simulink model "sys_PID"  (R2021a)
settings: Solver=FixedStepAuto  StartTime=0.0  StopTime=500  FixedStep=0.02  RelTol=1e-3
libraries: sharedutil x5, simulink x3, aerolibutil x1
(part 1 of 2)
settings Model: Creator=frede  LastModifiedBy=frede
settings DataIOCC: ReturnWorkspaceOutputs=off

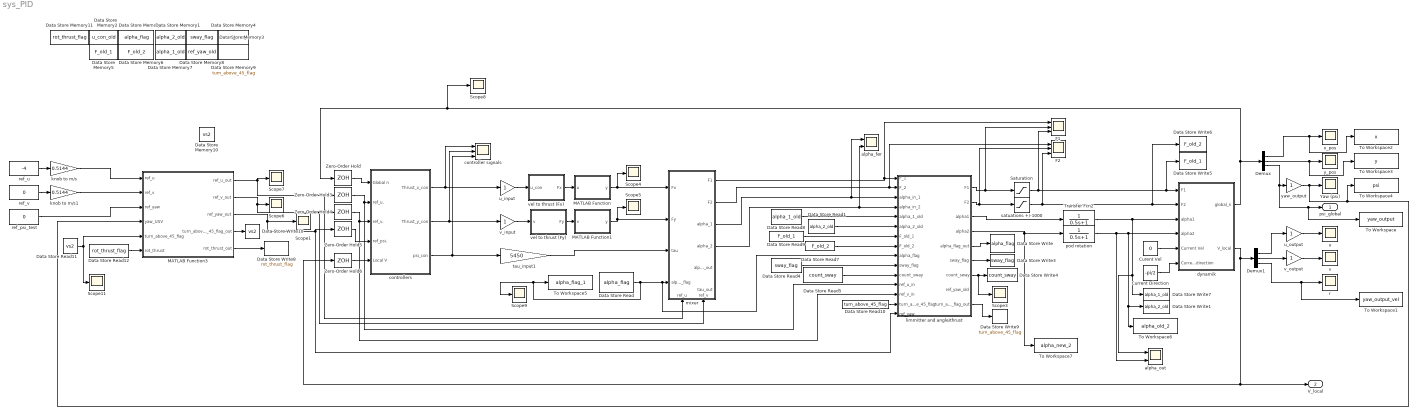
== system sys_PID ==
  Curent Vel : Constant  Value=0
  Current Direction : Constant  Value=-pi/2
  Data Store Memory : DataStoreMemory  DataStoreName=alpha_flag  ReadBeforeWriteMsg=warning  WriteAfterWriteMsg=warning  WriteAfterReadMsg=warning  ShowAdditionalParam=off
  Data Store Memory1 : DataStoreMemory  DataStoreName=alpha_2_old  ReadBeforeWriteMsg=warning  WriteAfterWriteMsg=warning  WriteAfterReadMsg=warning  ShowAdditionalParam=off
  Data Store Memory10 : DataStoreMemory  DataStoreName=vs2  ReadBeforeWriteMsg=warning  WriteAfterWriteMsg=warning  WriteAfterReadMsg=warning  ShowAdditionalParam=off
  Data Store Memory11 : DataStoreMemory  DataStoreName=rot_thrust_flag  ReadBeforeWriteMsg=warning  WriteAfterWriteMsg=warning  WriteAfterReadMsg=warning  ShowAdditionalParam=off
  Data Store Memory2 : DataStoreMemory  DataStoreName=u_con_old  ReadBeforeWriteMsg=warning  WriteAfterWriteMsg=warning  WriteAfterReadMsg=warning  ShowAdditionalParam=off
  Data Store Memory3 : DataStoreMemory  DataStoreName=sway_flag  ReadBeforeWriteMsg=warning  WriteAfterWriteMsg=warning  WriteAfterReadMsg=warning  ShowAdditionalParam=off
  Data Store Memory4 : DataStoreMemory  DataStoreName=count_sway  ReadBeforeWriteMsg=warning  WriteAfterWriteMsg=warning  WriteAfterReadMsg=warning  ShowAdditionalParam=off
  Data Store Memory5 : DataStoreMemory  DataStoreName=F_old_1  ReadBeforeWriteMsg=warning  WriteAfterWriteMsg=warning  WriteAfterReadMsg=warning  ShowAdditionalParam=off
  Data Store Memory6 : DataStoreMemory  DataStoreName=F_old_2  ReadBeforeWriteMsg=warning  WriteAfterWriteMsg=warning  WriteAfterReadMsg=warning  ShowAdditionalParam=off
  Data Store Memory7 : DataStoreMemory  DataStoreName=alpha_1_old  ReadBeforeWriteMsg=warning  WriteAfterWriteMsg=warning  WriteAfterReadMsg=warning  ShowAdditionalParam=off
  Data Store Memory8 : DataStoreMemory  DataStoreName=ref_yaw_old  ReadBeforeWriteMsg=warning  WriteAfterWriteMsg=warning  WriteAfterReadMsg=warning  ShowAdditionalParam=off
  Data Store Memory9 : DataStoreMemory  DataStoreName=turn_above_45_flag  ReadBeforeWriteMsg=warning  WriteAfterWriteMsg=warning  WriteAfterReadMsg=warning  ShowAdditionalParam=off
  Data Store Read : DataStoreRead  DataStoreName=alpha_flag  IndexOptions=Index vector (dialog)  Indices=1  OutputSizes=1
  Data Store Read1 : DataStoreRead  DataStoreName=alpha_2_old  IndexOptions=Index vector (dialog)  Indices=1  OutputSizes=1
  Data Store Read10 : DataStoreRead  DataStoreName=turn_above_45_flag  IndexOptions=Index vector (dialog)  Indices=1  OutputSizes=1
  Data Store Read11 : DataStoreRead  DataStoreName=vs2  IndexOptions=Index vector (dialog)  Indices=1  OutputSizes=1
  Data Store Read12 : DataStoreRead  DataStoreName=rot_thrust_flag  IndexOptions=Index vector (dialog)  Indices=1  OutputSizes=1
  Data Store Read4 : DataStoreRead  DataStoreName=sway_flag  IndexOptions=Index vector (dialog)  Indices=1  OutputSizes=1
  Data Store Read5 : DataStoreRead  DataStoreName=count_sway  IndexOptions=Index vector (dialog)  Indices=1  OutputSizes=1
  Data Store Read7 : DataStoreRead  DataStoreName=F_old_2  IndexOptions=Index vector (dialog)  Indices=1  OutputSizes=1
  Data Store Read8 : DataStoreRead  DataStoreName=alpha_1_old  IndexOptions=Index vector (dialog)  Indices=1  OutputSizes=1
  Data Store Read9 : DataStoreRead  DataStoreName=F_old_1  IndexOptions=Index vector (dialog)  Indices=1  OutputSizes=1
  Data Store Write : DataStoreWrite  DataStoreName=alpha_flag  IndexOptions=Index vector (dialog)  Indices=1  OutputSizes=1
  Data Store Write1 : DataStoreWrite  DataStoreName=alpha_2_old  IndexOptions=Index vector (dialog)  Indices=1  OutputSizes=1
  Data Store Write10 : DataStoreWrite  DataStoreName=vs2  IndexOptions=Index vector (dialog)  Indices=1  OutputSizes=1
  Data Store Write3 : DataStoreWrite  DataStoreName=sway_flag  IndexOptions=Index vector (dialog)  Indices=1  OutputSizes=1
  Data Store Write4 : DataStoreWrite  DataStoreName=count_sway  IndexOptions=Index vector (dialog)  Indices=1  OutputSizes=1
  Data Store Write5 : DataStoreWrite  DataStoreName=F_old_1  IndexOptions=Index vector (dialog)  Indices=1  OutputSizes=1
  Data Store Write6 : DataStoreWrite  DataStoreName=F_old_2  IndexOptions=Index vector (dialog)  Indices=1  OutputSizes=1
  Data Store Write7 : DataStoreWrite  DataStoreName=alpha_1_old  IndexOptions=Index vector (dialog)  Indices=1  OutputSizes=1
  Data Store Write8 : DataStoreWrite  DataStoreName=rot_thrust_flag  IndexOptions=Index vector (dialog)  Indices=1  OutputSizes=1
  Data Store Write9 : DataStoreWrite  DataStoreName=turn_above_45_flag  IndexOptions=Index vector (dialog)  Indices=1  OutputSizes=1
  Demux : Demux  Outputs=3
  Demux1 : Demux  Outputs=3
  F1 : Scope  NumInputPorts=3
  F2 : Scope  NumInputPorts=3
  MATLAB Function : MATLAB Function  TreatAsAtomicUnit=on
  MATLAB Function1 : MATLAB Function  TreatAsAtomicUnit=on
  MATLAB Function3 : MATLAB Function  TreatAsAtomicUnit=on
  Saturation : Saturate  UpperLimit=1000  LowerLimit=-1000
  Scope{1,3..9,11} (9 alike) : Scope
  To Workspace : ToWorkspace  VariableName=yaw_output  SaveFormat=Timeseries  SampleTime=-1
  To Workspace1 : ToWorkspace  VariableName=yaw_output_vel  SaveFormat=Timeseries  SampleTime=-1
  To Workspace2 : ToWorkspace  VariableName=x  SaveFormat=Timeseries  SampleTime=-1
  To Workspace3 : ToWorkspace  VariableName=y  SaveFormat=Timeseries  SampleTime=-1
  To Workspace4 : ToWorkspace  VariableName=psi  SaveFormat=Timeseries  SampleTime=-1
  To Workspace5 : ToWorkspace  VariableName=alpha_flag_1  SaveFormat=Timeseries  SampleTime=-1
  To Workspace6 : ToWorkspace  VariableName=alpha_old_2  SaveFormat=Timeseries  SampleTime=-1
  To Workspace7 : ToWorkspace  VariableName=alpha_new_2  SaveFormat=Timeseries  SampleTime=-1
  Transfer Fcn2 : TransferFcn  Denominator=[0.5 1]
  Yaw (psi) : Scope
  Zero-Order Hold{,3..6} (5 alike) : ZeroOrderHold  SampleTime=1/10
  alpha_før : Scope  NumInputPorts=2
  alpha_out : Scope  NumInputPorts=2
  controller signals : Scope  NumInputPorts=3
  controllers : Subsystem
  dynamik : Subsystem
  knob to m/s : Gain  Gain=0.5144
  knob to m/s1 : Gain  Gain=0.5144
  "limmitter and angle/thrust " : MATLAB Function  TreatAsAtomicUnit=on
  mixer : Subsystem
      settings: PortSchema="{\"entries\":[{\"content\":{\"sides\":[{\"content\":{\"connectorIds\":[\"In1\",\"In2\",\"In3\",\"In4\"]},\"type\":\"ConnectorPlacement.EquallySpacedRectSide\",\"uuid\":\"7188d02b-cfcc-47db-af94-18894173419c\"},{\"content\":{\"connectorIds\":[\"Out1\",\"Out2\",\"Out3\",\"Out4\",\"Out5\",\"Out6\"],\"side\":\"RIGHT\"},\"type\":\"ConnectorPlacement.EquallySpacedRectSide\",\"uuid\":\"02945fdb-bbe4-4a20-85bf-b896b72802e6\"},{\"content\":{\"connectorIds\":[],\"side\":\"TOP\"},\"type\":\"ConnectorPlacement.EquallySpacedRectSide\",\"uuid\":\"f10c450a-087c-46ba-bf6c-a28873fc7004\"},{\"content\":{\"connectorIds\":[\"In5\",\"In6\"],\"side\":\"BOTTOM\"},\"type\":\"ConnectorPlacement.EquallySpacedRectSide\",\"uuid\":\"e6b9d579-da5b-4e58-b3fd-82de45e53b4e\"}]},\"type\":\"ConnectorPlacement.EquallySpacedConnector\",\"uuid\":\"11fe65e6-3ea5-4662-a95f-67184bab7731\"}],\"packageUris\":[\"http://schema.mathworks.com/mf0/Connector/R2020b\"],\"version\":\"1.0\"}"
  pod rotation : TransferFcn  Denominator=[0.5 1]
  r : Scope
  ref_psi_test : Constant  Value=0
  ref_u : Constant  Value=-4
  ref_v : Constant  Value=0
  "satuations +/-1000 " : Saturate  UpperLimit=1000  LowerLimit=-1000
  tau_input1 : Gain  Gain=5450
  u : Scope
  u_input : Gain
  u_output : Gain
  v : Scope
  v_input : Gain
  v_output : Gain
  vel to thrust (Fx) : MATLAB Function  TreatAsAtomicUnit=on
  vel to thrust (Fy) : MATLAB Function  TreatAsAtomicUnit=on
  x_pos : Scope
  y_pos : Scope
  yaw_output : Gain
  psi_global : Outport
  V_local : Outport  Port=2
  wires:
  u_output/1 -> u/1
  vel to thrust (Fx)/1(Fx) -> MATLAB Function/1(u)
  Demux1/3 -> To Workspace1/1, r/1
  "limmitter and angle/thrust "/2(F2) -> "satuations +/-1000 "/1, F2/2
  mixer/1(F1) -> F1/1, "limmitter and angle/thrust "/1(F_1)
  v_input/1 -> vel to thrust (Fy)/1(v)
  pod rotation/1 -> dynamik/4(alpha2), To Workspace6/1, Data Store Write1/1, alpha_out/2
  mixer/4(alpha_2) -> alpha_før/2, "limmitter and angle/thrust "/4(alpha_in_2)
  Demux1/2 -> v_output/1
  mixer/2(F2) -> F2/1, "limmitter and angle/thrust "/2(F_2)
  "limmitter and angle/thrust "/3(alpha1) -> Transfer Fcn2/1
  u_input/1 -> vel to thrust (Fx)/1(u_con)
  MATLAB Function1/1(y) -> Scope5/1, mixer/2(Fy)
  mixer/3(alpha_1) -> alpha_før/1, "limmitter and angle/thrust "/3(alpha_in_1)
  "limmitter and angle/thrust "/1(F1) -> F1/2, Saturation/1
  Demux/2 -> To Workspace3/1, y_pos/1
  "satuations +/-1000 "/1 -> Data Store Write6/1, dynamik/2(F2), F2/3
  Demux1/1 -> u_output/1
  Transfer Fcn2/1 -> Data Store Write7/1, alpha_out/1, dynamik/3(alpha1)
  dynamik/1(global_n) -> Scope8/1, Zero-Order Hold/1, Demux/1
  "limmitter and angle/thrust "/4(alpha2) -> To Workspace7/1, pod rotation/1
  Demux/1 -> To Workspace2/1, x_pos/1
  v_output/1 -> v/1
  Saturation/1 -> Data Store Write5/1, dynamik/1(F1), F1/3
  ref_v/1 -> knob to m/s1/1
  Demux/3 -> yaw_output/1, To Workspace/1, psi_global/1
  MATLAB Function/1(y) -> Scope4/1, mixer/1(Fx)
  yaw_output/1 -> MATLAB Function3/4(yaw_USV), To Workspace4/1, Yaw (psi)/1
  vel to thrust (Fy)/1(Fy) -> MATLAB Function1/1(v)
  MATLAB Function3/3(ref_yaw_out) -> Zero-Order Hold5/1, "limmitter and angle/thrust "/15(ref_yaw), Scope1/1
  Curent Vel/1 -> dynamik/5(Current Vel)
  Current Direction/1 -> dynamik/6(Current direction)
  ref_u/1 -> knob to m/s/1
  MATLAB Function3/2(ref_v_out) -> Zero-Order Hold4/1, mixer/6(ref_v), Scope6/1
  "limmitter and angle/thrust "/5(alpha_flag_out) -> Data Store Write/1
  Data Store Read1/1 -> "limmitter and angle/thrust "/6(alpha_2_old)
  Data Store Read/1 -> Scope9/1, To Workspace5/1, "limmitter and angle/thrust "/9(alpha_flag), mixer/4(alpha_flag)
  Zero-Order Hold/1 -> controllers/1(Global n)
  MATLAB Function3/1(ref_u_out) -> Scope7/1, Zero-Order Hold3/1, mixer/5(ref_u)
  dynamik/2(V_local) -> Zero-Order Hold6/1, V_local/1, Demux1/1
  Zero-Order Hold3/1 -> "limmitter and angle/thrust "/12(ref_u_in), controllers/2(ref_u.)
  Zero-Order Hold4/1 -> controllers/3(ref_v.), "limmitter and angle/thrust "/13(ref_v_in)
  Zero-Order Hold5/1 -> controllers/4(ref_psi.)
  Zero-Order Hold6/1 -> controllers/5(Local V)
  "limmitter and angle/thrust "/6(sway_flag) -> Data Store Write3/1
  Data Store Read5/1 -> "limmitter and angle/thrust "/11("count_sway ")
  tau_input1/1 -> mixer/3(tau)
  Data Store Read8/1 -> "limmitter and angle/thrust "/5(alpha_1_old)
  Data Store Read7/1 -> "limmitter and angle/thrust "/8(F_old_2)
  Data Store Read9/1 -> "limmitter and angle/thrust "/7(F_old_1)
  Data Store Read4/1 -> "limmitter and angle/thrust "/10("sway_flag ")
  "limmitter and angle/thrust "/7(count_sway) -> Scope3/1, Data Store Write4/1
  Data Store Read10/1 -> "limmitter and angle/thrust "/14(turn_above_45_flag)
  "limmitter and angle/thrust "/9(turn_above_45_flag_out) -> Data Store Write9/1
  MATLAB Function3/4(turn_above_45_flag_out) -> Data Store Write10/1
  Data Store Read11/1 -> Scope11/1, MATLAB Function3/5(turn_above_45_flag)
  controllers/2(Thrust_y_con) -> v_input/1, controller signals/2
  controllers/1(Thrust_x_con) -> controller signals/1, u_input/1
  controllers/3(psi_con) -> tau_input1/1, controller signals/3
  Data Store Read12/1 -> MATLAB Function3/6(rot_thrust)
  MATLAB Function3/5(rot_thrust_out) -> Data Store Write8/1
  knob to m/s/1 -> MATLAB Function3/1(ref_u)
  knob to m/s1/1 -> MATLAB Function3/2(ref_v)
  ref_psi_test/1 -> MATLAB Function3/3(ref_yaw)

== system sys_PID/controllers ==
  Global n : Inport
  ref_u. : Inport  Port=2
  ref_v. : Inport  Port=3
  ref_psi. : Inport  Port=4
  Local V : Inport  Port=5
  PIDs : Subsystem
  Thrust_x_con : Outport
  Thrust_y_con : Outport  Port=2
  psi_con : Outport  Port=3
  wires:
  Global n/1 -> PIDs/1(n)
  ref_v./1 -> PIDs/4(ref_v_)
  PIDs/3(diff_psi) -> psi_con/1
  PIDs/1(sig_u) -> Thrust_x_con/1
  PIDs/2(sig_v) -> Thrust_y_con/1
  ref_u./1 -> PIDs/2(ref_u_)
  Local V/1 -> PIDs/3(V)
  ref_psi./1 -> PIDs/5(ref_psi_)

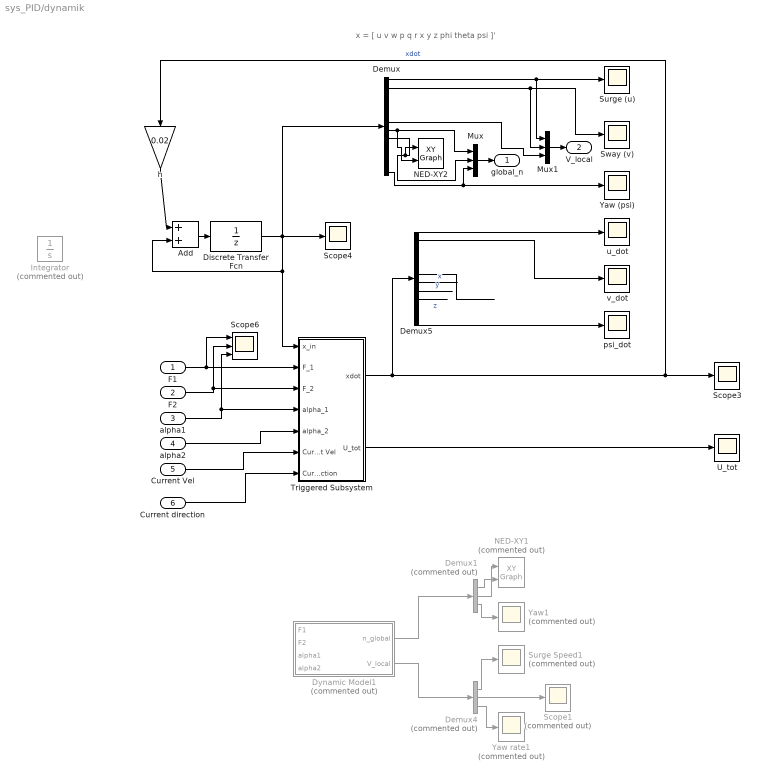
== system sys_PID/dynamik ==
  note: x = [ u v w p q r x y z phi theta psi ]'
  F1 : Inport
  F2 : Inport  Port=2
  alpha1 : Inport  Port=3
  alpha2 : Inport  Port=4
  Current Vel : Inport  Port=5
  Current direction : Inport  Port=6
  Add : Sum
  Demux : Demux  Outputs=12
  Demux1 : Demux  Commented=on  Outputs=3
  Demux4 : Demux  Commented=on  Outputs=3
  Demux5 : Demux  Outputs=12
  Discrete Transfer Fcn : DiscreteTransferFcn  Denominator=[ 1 0]  SampleTime=0.02
  Dynamic Model1 : Subsystem  Commented=on
  Integrator : Integrator  Commented=on
  Mux : Mux  Inputs=3
  Mux1 : Mux  Inputs=3
  NED-XY1 : simulink/Sinks/XY Graph  Commented=on  xmin=-1000  xmax=1000  ymin=-1000  ymax=1000  st=-1
  NED-XY2 : simulink/Sinks/XY Graph  xmin=-1000  xmax=1000  ymin=-1000  ymax=1000  st=-1
  Scope1 : Scope  Commented=on
  Scope3 : Scope
  Scope4 : Scope
  Scope6 : Scope  NumInputPorts=3
  Surge (u) : Scope
  Surge Speed1 : Scope  Commented=on
  Sway (v) : Scope
  Triggered Subsystem : Subsystem  TreatAsAtomicUnit=on
  U_tot : Scope
  Yaw (psi) : Scope
  Yaw rate1 : Scope  Commented=on
  Yaw1 : Scope  Commented=on
  h : Gain  Gain=0.02
  psi_dot : Scope
  u_dot : Scope
  v_dot : Scope
  global_n : Outport
  V_local : Outport  Port=2
  wires:
  Demux1/3 -> Yaw1/1
  Demux4/3 -> Yaw rate1/1
  Demux1/2 -> NED-XY1/1
  Demux4/2 -> Scope1/1
  Demux1/1 -> NED-XY1/2
  Demux4/1 -> Surge Speed1/1
  Dynamic Model1/1(n_global) -> Demux1/1
  Dynamic Model1/2(V_local) -> Demux4/1
  F1/1 -> Scope6/1, Triggered Subsystem/2(F_1)
  F2/1 -> Scope6/2, Triggered Subsystem/3(F_2)
  alpha1/1 -> Scope6/3, Triggered Subsystem/4(alpha_1)
  alpha2/1 -> Triggered Subsystem/5(alpha_2)
  h/1 -> Add/1
  Add/1 -> Discrete Transfer Fcn/1
  Triggered Subsystem/1(xdot) -> Demux5/1, Scope3/1, h/1  "xdot"
  Triggered Subsystem/2(U_tot) -> U_tot/1
  Demux/8 -> Mux/2, NED-XY2/1
  Demux/7 -> NED-XY2/2, Mux/1
  Discrete Transfer Fcn/1 -> Scope4/1, Demux/1, Add/2, Triggered Subsystem/1(x_in)
  Demux/1 -> Surge (u)/1, Mux1/1
  Demux/12 -> Mux/3, Yaw (psi)/1
  Demux/2 -> Mux1/2, Sway (v)/1
  Mux/1 -> global_n/1
  Demux5/12 -> psi_dot/1
  Demux5/2 -> v_dot/1
  Demux5/1 -> u_dot/1
  Demux5/9 -> ?  "z"
  Demux5/7 -> ?  "x"
  Demux5/8 -> ?  "y"
  Mux1/1 -> V_local/1
  Demux5/6 -> ?
  Demux/6 -> Mux1/3
  Current Vel/1 -> Triggered Subsystem/6(Current Vel)
  Current direction/1 -> Triggered Subsystem/7(Current Direction)

== system sys_PID/mixer ==
  Fx : Inport
  Fy : Inport  Port=2
  tau : Inport  Port=3
  alpha_flag : Inport  Port=4
  ref_u : Inport  Port=5
  ref_v : Inport  Port=6
  MATLAB Function : MATLAB Function  TreatAsAtomicUnit=on
  d : Constant  Value=1.3395
  F1 : Outport
  F2 : Outport  Port=2
  alpha_1 : Outport  Port=3
  alpha_2 : Outport  Port=4
  alpha_flag_out : Outport  Port=5
  tau_out : Outport  Port=6
  wires:
  d/1 -> MATLAB Function/4(d)
  MATLAB Function/1(F_1) -> F1/1
  Fx/1 -> MATLAB Function/1(F_x)
  Fy/1 -> MATLAB Function/2(F_y)
  tau/1 -> MATLAB Function/3(tau)
  MATLAB Function/2(F_2) -> F2/1
  MATLAB Function/3(alpha1) -> alpha_1/1
  MATLAB Function/4(alpha2) -> alpha_2/1
  alpha_flag/1 -> MATLAB Function/5(alpha_flag)
  MATLAB Function/5(alpha_flag_out) -> alpha_flag_out/1
  ref_u/1 -> MATLAB Function/7(ref_u)
  ref_v/1 -> MATLAB Function/8(ref_v)
  MATLAB Function/6(tau_out) -> tau_out/1

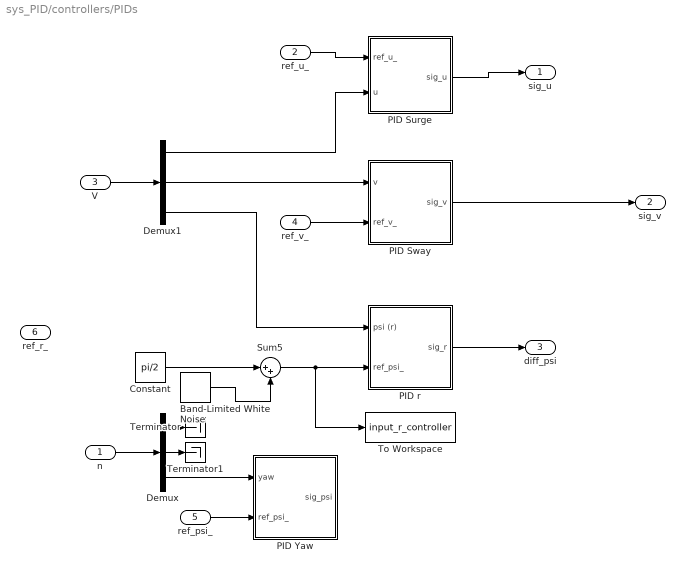
== system sys_PID/controllers/PIDs ==
  n : Inport
  ref_u_ : Inport  Port=2
  V : Inport  Port=3
  ref_v_ : Inport  Port=4
  ref_psi_ : Inport  Port=5
  ref_r_ : Inport  Port=6
  Band-Limited White Noise : simulink/Sources/Band-Limited White Noise  Cov=[0.01]  Ts=0.1  seed=[23341]
  Constant : Constant  Value=pi/2
  Demux : Demux  Outputs=3
  Demux1 : Demux  Outputs=3
  PID Surge : Subsystem
  PID Sway : Subsystem
  PID Yaw : Subsystem
  PID r : Subsystem
  Sum5 : Sum  Inputs=|++
  Terminator : Terminator
  Terminator1 : Terminator
  To Workspace : ToWorkspace  VariableName=input_r_controller  SaveFormat=Timeseries  SampleTime=-1
  sig_u : Outport
  sig_v : Outport  Port=2
  diff_psi : Outport  Port=3
  wires:
  n/1 -> Demux/1
  Demux/3 -> PID Yaw/1(yaw)
  Demux/1 -> Terminator/1
  Demux/2 -> Terminator1/1
  Demux1/3 -> PID r/1(psi (r))
  V/1 -> Demux1/1
  ref_u_/1 -> PID Surge/1(ref_u_)
  Demux1/1 -> PID Surge/2(u)
  Demux1/2 -> PID Sway/1(v)
  ref_v_/1 -> PID Sway/2(ref_v_)
  Band-Limited White Noise/1 -> Sum5/2
  Constant/1 -> Sum5/1
  PID Sway/1(sig_v) -> sig_v/1
  PID Surge/1(sig_u) -> sig_u/1
  PID r/1(sig_r) -> diff_psi/1
  ref_psi_/1 -> PID Yaw/2(ref_psi_)
  Sum5/1 -> To Workspace/1, PID r/2(ref_psi_)

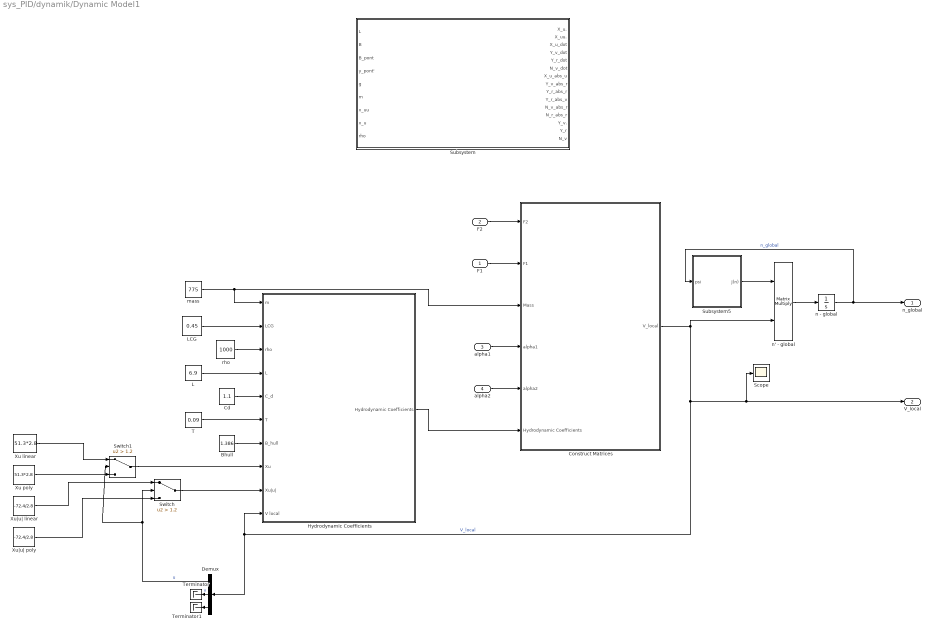
== system sys_PID/dynamik/Dynamic Model1 ==
  F1 : Inport
  F2 : Inport  Port=2
  alpha1 : Inport  Port=3
  alpha2 : Inport  Port=4
  "Bhull " : Constant  Value=1.386
  Cd : Constant  Value=1.1
  Construct Matrices : Subsystem
  Demux : Demux  Outputs=3
  Hydrodynamic Coefficients : Subsystem
  L : Constant  Value=6.9
  LCG : Constant  Value=0.45
  Scope : Scope
  Subsystem : Subsystem
  Subsystem5 : Subsystem
  Switch : Switch  Criteria=u2 > Threshold  Threshold=1.2
  Switch1 : Switch  Criteria=u2 > Threshold  Threshold=1.2
  T : Constant  Value=0.09
  Terminator : Terminator
  Terminator1 : Terminator
  Xu linear : Constant  Value=51.3*2.8
  Xu poly : Constant  Value=51.3*2.8
  Xu|u| linear : Constant  Value=-72.4/2.8
  Xu|u| poly : Constant  Value=-72.4/2.8
  mass : Constant  Value=775
  n - global : Integrator  InitialCondition=[0 0 0]
  n' - global : Product  Multiplication=Matrix(*)
  rho : Constant  Value=1000
  n_global : Outport  VectorParamsAs1DForOutWhenUnconnected=off
  V_local : Outport  Port=2  VectorParamsAs1DForOutWhenUnconnected=off
  wires:
  n - global/1 -> Subsystem5/1(psi), n_global/1  "n_global"
  Cd/1 -> Hydrodynamic Coefficients/5(C_d)
  Construct Matrices/1(V_local) -> n' - global/2, Demux/1, Hydrodynamic Coefficients/10(V local), Scope/1, V_local/1  "V_local"
  n' - global/1 -> n - global/1
  Subsystem5/1(J(n)) -> n' - global/1
  rho/1 -> Hydrodynamic Coefficients/3(rho)
  L/1 -> Hydrodynamic Coefficients/4(L)
  F2/1 -> Construct Matrices/1(F2)
  F1/1 -> Construct Matrices/2(F1)
  mass/1 -> Hydrodynamic Coefficients/1(m), Construct Matrices/3("Mass ")
  Hydrodynamic Coefficients/1("Hydrodynamic Coefficients ") -> Construct Matrices/6(Hydrodynamic Coefficients)
  T/1 -> Hydrodynamic Coefficients/6(T)
  "Bhull "/1 -> Hydrodynamic Coefficients/7(B_hull)
  Switch/1 -> Hydrodynamic Coefficients/9(Xu|u|)
  LCG/1 -> Hydrodynamic Coefficients/2(LCG)
  Demux/1 -> Switch1/2, Switch/2  "u"
  Xu|u| poly/1 -> Switch/3
  Xu|u| linear/1 -> Switch/1
  Switch1/1 -> Hydrodynamic Coefficients/8(Xu)
  Xu poly/1 -> Switch1/3
  Xu linear/1 -> Switch1/1
  Demux/3 -> Terminator1/1
  Demux/2 -> Terminator/1  "v"
  alpha1/1 -> Construct Matrices/4(alpha1)
  alpha2/1 -> Construct Matrices/5(alpha2)

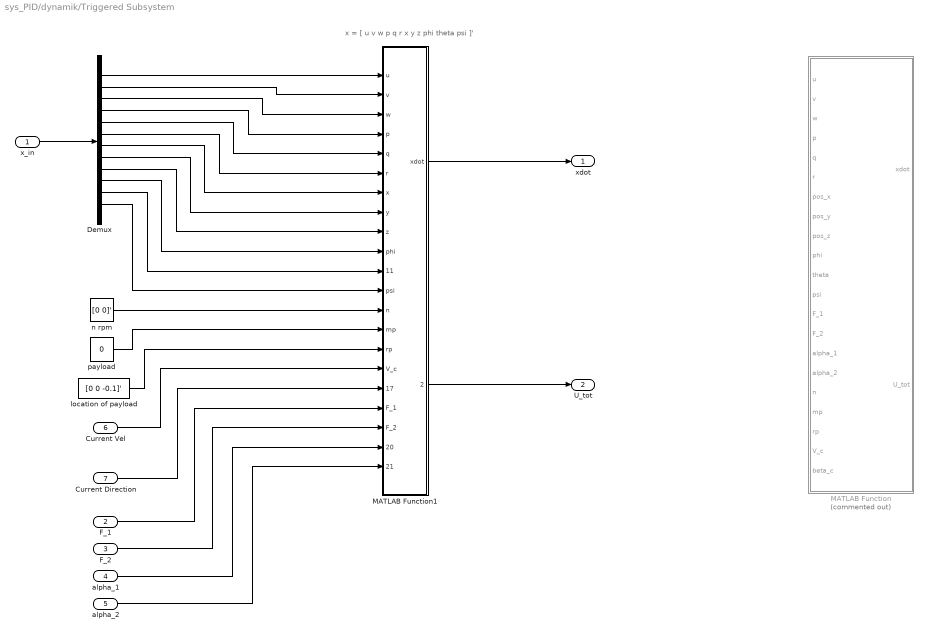
== system sys_PID/dynamik/Triggered Subsystem ==
  note: x = [ u v w p q r x y z phi theta psi ]'
  x_in : Inport
  F_1 : Inport  Port=2
  F_2 : Inport  Port=3
  alpha_1 : Inport  Port=4
  alpha_2 : Inport  Port=5
  Current Vel : Inport  Port=6
  Current Direction : Inport  Port=7
  Demux : Demux  Outputs=12
  MATLAB Function : MATLAB Function  Commented=on  TreatAsAtomicUnit=on
  MATLAB Function1 : MATLAB Function  TreatAsAtomicUnit=on
  location of payload : Constant  Value=[0 0 -0.1]'
  n rpm : Constant  Value=[0 0]'
  payload : Constant  Value=0
  xdot : Outport
  U_tot : Outport  Port=2
  wires:
  F_1/1 -> MATLAB Function1/18(F_1)
  F_2/1 -> MATLAB Function1/19(F_2)
  alpha_1/1 -> MATLAB Function1/20(alpha_1)
  alpha_2/1 -> MATLAB Function1/21(alpha_2)
  location of payload/1 -> MATLAB Function1/15(rp)
  payload/1 -> MATLAB Function1/14(mp)
  Current Vel/1 -> MATLAB Function1/16(V_c)
  Current Direction/1 -> MATLAB Function1/17(beta_c)
  n rpm/1 -> MATLAB Function1/13(n)
  x_in/1 -> Demux/1
  MATLAB Function1/2(U_tot) -> U_tot/1
  MATLAB Function1/1(xdot) -> xdot/1
  Demux/1 -> MATLAB Function1/1(u)
  Demux/2 -> MATLAB Function1/2(v)
  Demux/3 -> MATLAB Function1/3(w)
  Demux/4 -> MATLAB Function1/4(p)
  Demux/5 -> MATLAB Function1/5(q)
  Demux/6 -> MATLAB Function1/6(r)
  Demux/7 -> MATLAB Function1/7(x)
  Demux/8 -> MATLAB Function1/8(y)
  Demux/9 -> MATLAB Function1/9(z)
  Demux/10 -> MATLAB Function1/10(phi)
  Demux/11 -> MATLAB Function1/11(theta)
  Demux/12 -> MATLAB Function1/12(psi)

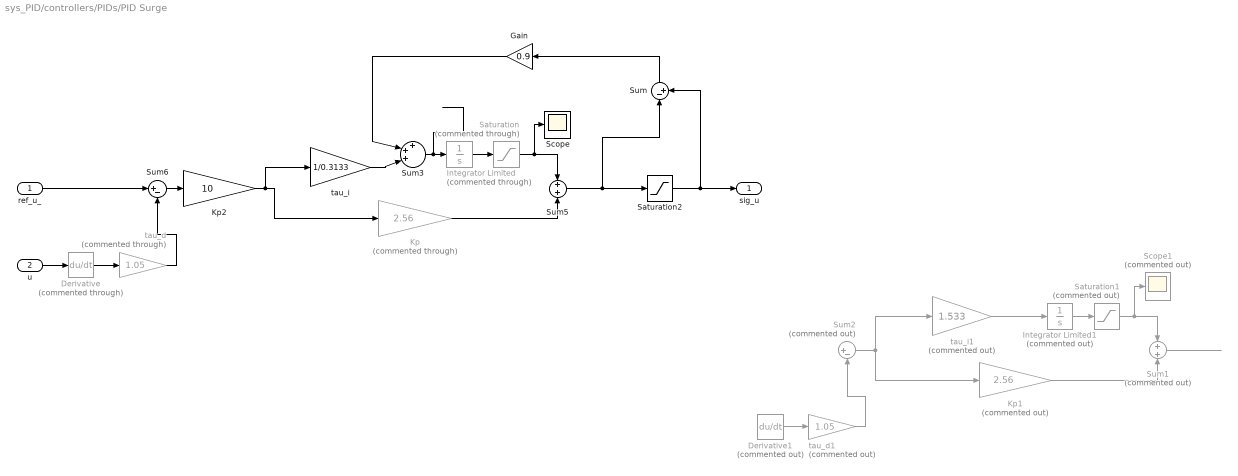
== system sys_PID/controllers/PIDs/PID Surge ==
  ref_u_ : Inport
  u : Inport  Port=2
  Derivative : Derivative  Commented=through
  Derivative1 : Derivative  Commented=on
  Gain : Gain  Gain=0.9
  Integrator Limited : Integrator  Commented=through  LimitOutput=on  UpperSaturationLimit=1  LowerSaturationLimit=-1
  Integrator Limited1 : Integrator  Commented=on  LimitOutput=on  UpperSaturationLimit=1  LowerSaturationLimit=-1
  Kp : Gain  Commented=through  Gain=2.56
  Kp1 : Gain  Commented=on  Gain=2.56
  Kp2 : Gain  Gain=10
  Saturation : Saturate  Commented=through  UpperLimit=5  LowerLimit=-5
  Saturation1 : Saturate  Commented=on  UpperLimit=5  LowerLimit=-5
  Saturation2 : Saturate  UpperLimit=4  LowerLimit=-4
  Scope : Scope
  Scope1 : Scope  Commented=on
  Sum : Sum  Inputs=|-+
  Sum1 : Sum  Commented=on
  Sum2 : Sum  Commented=on  Inputs=|+-
  Sum3 : Sum  Inputs=+++|
  Sum5 : Sum
  Sum6 : Sum  Inputs=|+-
  tau_d : Gain  Commented=through  Gain=1.05
  tau_d1 : Gain  Commented=on  Gain=1.05
  tau_i : Gain  Gain=1/0.3133
  tau_i1 : Gain  Commented=on  Gain=1.533
  sig_u : Outport
  wires:
  ref_u_/1 -> Sum6/1
  tau_d/1 -> Sum6/2
  Derivative/1 -> tau_d/1
  Kp/1 -> Sum5/2
  Sum6/1 -> Kp2/1
  u/1 -> Derivative/1
  tau_i/1 -> Sum3/3
  Integrator Limited/1 -> Saturation/1
  Saturation/1 -> Sum5/1, Scope/1
  ? -> Sum2/1
  Sum2/1 -> tau_i1/1, Kp1/1
  Kp1/1 -> Sum1/2
  Derivative1/1 -> tau_d1/1
  Saturation1/1 -> Sum1/1, Scope1/1
  ? -> Derivative1/1
  tau_d1/1 -> Sum2/2
  Integrator Limited1/1 -> Saturation1/1
  Sum1/1 -> ?
  tau_i1/1 -> Integrator Limited1/1
  Sum5/1 -> Saturation2/1, Sum/1
  Saturation2/1 -> sig_u/1, Sum/2
  Sum/1 -> Gain/1
  Gain/1 -> Sum3/2
  Kp2/1 -> tau_i/1, Kp/1
  Sum3/1 -> Integrator Limited/1
  ? -> Sum3/1

== system sys_PID/controllers/PIDs/PID Sway ==
  v : Inport
  ref_v_ : Inport  Port=2
  Derivative1 : Derivative  Commented=through
  Integrator Limited : Integrator  LimitOutput=on  UpperSaturationLimit=1  LowerSaturationLimit=-1
  Kp : Gain  Gain=2
  Saturation : Saturate  UpperLimit=1  LowerLimit=-1
  Scope : Scope
  Sum7 : Sum
  Sum8 : Sum  Inputs=|+-
  tau_d1 : Gain
  tau_i : Gain  Gain=0.5
  sig_v : Outport
  wires:
  Sum8/1 -> tau_i/1, Kp/1
  Kp/1 -> Sum7/2
  ref_v_/1 -> Sum8/1
  Integrator Limited/1 -> Saturation/1
  Derivative1/1 -> tau_d1/1
  Sum7/1 -> sig_v/1
  tau_d1/1 -> Sum8/2
  v/1 -> Derivative1/1
  tau_i/1 -> Integrator Limited/1
  Saturation/1 -> Scope/1, Sum7/1

== system sys_PID/controllers/PIDs/PID Yaw ==
  yaw : Inport
  ref_psi_ : Inport  Port=2
  Derivative1 : Derivative  Commented=through
  Derivative2 : Derivative  Commented=through
  Integrator1 : Integrator
  Kp : Gain  Gain=0.1654
  Sum7 : Sum  Inputs=+++
  Sum8 : Sum  Inputs=|+-
  tau_d : Gain  Commented=through  Gain=10000
  tau_d1 : Gain  Commented=through  Gain=0.001
  tau_i : Gain  Gain=0
  sig_psi : Outport
  wires:
  Sum8/1 -> Kp/1, Integrator1/1
  Integrator1/1 -> tau_i/1
  Kp/1 -> Sum7/2
  ref_psi_/1 -> Sum8/1
  tau_i/1 -> Sum7/1
  Derivative1/1 -> tau_d/1
  Sum7/1 -> sig_psi/1
  tau_d/1 -> Sum8/2
  yaw/1 -> Derivative1/1
  Derivative2/1 -> tau_d1/1
  tau_d1/1 -> Sum7/3

== system sys_PID/controllers/PIDs/PID r ==
  psi (r) : Inport
  ref_psi_ : Inport  Port=2
  Derivative1 : Derivative  Commented=through
  Integrator Limited : Integrator  LimitOutput=on  UpperSaturationLimit=0.2  LowerSaturationLimit=-0.2
  Kp : Gain  Commented=through  Gain=2
  Kp1 : Gain  Gain=1.2
  Saturation1 : Saturate  UpperLimit=10  LowerLimit=-10
  Sum7 : Sum
  Sum8 : Sum  Inputs=|+-
  tau_d : Gain
  tau_i : Gain  Gain=0.33
  sig_r : Outport
  wires:
  Sum8/1 -> Kp1/1
  Kp/1 -> Sum7/2
  ref_psi_/1 -> Sum8/1
  Integrator Limited/1 -> Saturation1/1
  Derivative1/1 -> tau_d/1
  Sum7/1 -> sig_r/1
  tau_d/1 -> Sum8/2
  psi (r)/1 -> Derivative1/1
  tau_i/1 -> Integrator Limited/1
  Kp1/1 -> Kp/1, tau_i/1
  Saturation1/1 -> Sum7/1

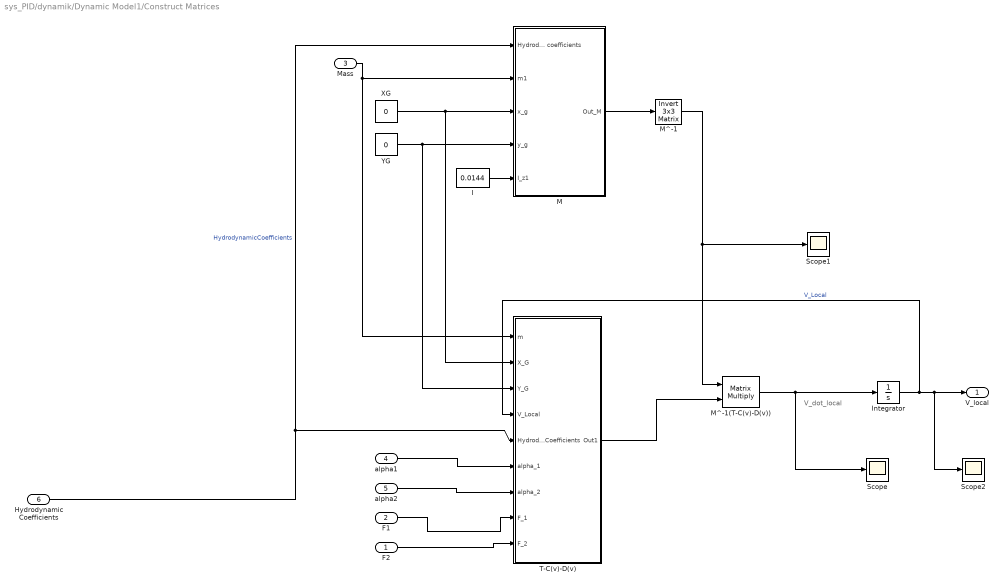
== system sys_PID/dynamik/Dynamic Model1/Construct Matrices ==
  note: V_dot_local
  F2 : Inport
  F1 : Inport  Port=2
  "Mass " : Inport  Port=3
  alpha1 : Inport  Port=4
  alpha2 : Inport  Port=5
  Hydrodynamic Coefficients : Inport  Port=6
  I : Constant  Value=0.0144
  Integrator : Integrator  InitialCondition=[0 0 0]
  M : Subsystem
  M^-1 : aerolibutil/Invert  3x3 Matrix
  M^-1(T-C(v)-D(v)) : Product  Multiplication=Matrix(*)
  Scope : Scope
  Scope1 : Scope
  Scope2 : Scope
  T-C(v)-D(v) : Subsystem
  XG : Constant  Value=0
  YG : Constant  Value=0
  V_local : Outport  VectorParamsAs1DForOutWhenUnconnected=off
  wires:
  Integrator/1 -> Scope2/1, V_local/1, T-C(v)-D(v)/4(V_Local)  "V_Local"
  M^-1(T-C(v)-D(v))/1 -> Scope/1, Integrator/1
  M/1(Out_M) -> M^-1/1
  Hydrodynamic Coefficients/1 -> M/1(Hydrodynamic coefficients), T-C(v)-D(v)/5(HydrodynamicCoefficients)  "HydrodynamicCoefficients"
  YG/1 -> M/4(y_g), T-C(v)-D(v)/3(Y_G)
  "Mass "/1 -> T-C(v)-D(v)/1(m), M/2(m1)
  XG/1 -> M/3(x_g), T-C(v)-D(v)/2(X_G)
  F1/1 -> T-C(v)-D(v)/8(F_1)
  F2/1 -> T-C(v)-D(v)/9(F_2)
  T-C(v)-D(v)/1(Out1) -> M^-1(T-C(v)-D(v))/2
  I/1 -> M/5(I_z1)
  alpha1/1 -> T-C(v)-D(v)/6(alpha_1)
  alpha2/1 -> T-C(v)-D(v)/7(alpha_2)
  M^-1/1 -> Scope1/1, M^-1(T-C(v)-D(v))/1

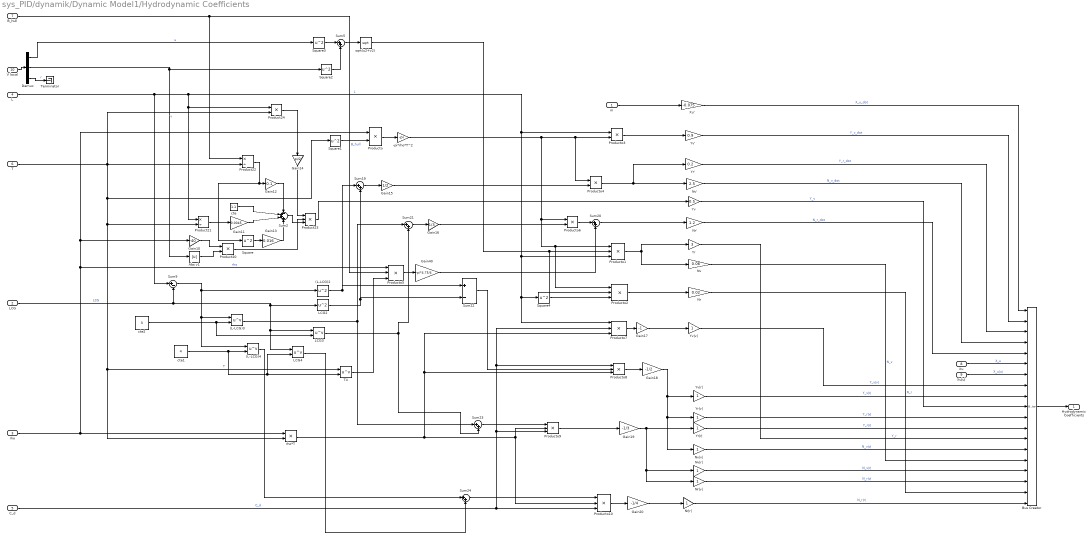
== system sys_PID/dynamik/Dynamic Model1/Hydrodynamic Coefficients ==
  m : Inport
  LCG : Inport  Port=2
  rho : Inport  Port=3
  L : Inport  Port=4
  C_d : Inport  Port=5
  T : Inport  Port=6
  B_hull : Inport  Port=7
  Xu : Inport  Port=8
  Xu|u| : Inport  Port=9
  V local : Inport  Port=10
  (L-LCG)2 : Math  Operator=square  SignedPower=on  SaturateOnIntegerOverflow=on
  (L-LCG)3 : Math  Operator=pow  SignedPower=on  SaturateOnIntegerOverflow=on
  (L-LCG)4 : Math  Operator=pow  SignedPower=on  SaturateOnIntegerOverflow=on
  -pi*rho*T^2 : Gain  Gain=-pi
  Abs v1 : Abs
  Bus Creator : BusCreator  Inputs=19
  Demux : Demux  Outputs=3
  Gain10 : Gain  Gain=-40
  Gain11 : Gain  Gain=0.0045
  Gain12 : Gain  Gain=0.1
  Gain13 : Gain  Gain=0.016
  Gain14 : Gain  Gain=pi/2
  Gain15 : Gain  Gain=1/2
  Gain16 : Gain  Gain=1/3
  Gain17 : Gain  Gain=-1
  Gain18 : Gain  Gain=-1/2
  Gain19 : Gain  Gain=-1/3
  Gain20 : Gain  Gain=-1/4
  Gain40 : Gain  Gain=-pi*4.75/4
  LCG2 : Math  Operator=square  SignedPower=on  SaturateOnIntegerOverflow=on
  LCG3 : Math  Operator=pow  SignedPower=on  SaturateOnIntegerOverflow=on
  LCG4 : Math  Operator=pow  SignedPower=on  SaturateOnIntegerOverflow=on
  Nr : Gain  Gain=0.02
  Nr' : Gain  Gain=1.2
  Nr|r| : Gain
  Nr|v| : Gain
  Nv : Gain  Gain=0.06
  Nv' : Gain  Gain=2.5
  Nv|r| : Gain
  Nv|v| : Gain
  Product20 : Product
  Product21 : Product  Inputs=*/
  Product22 : Product  Inputs=*/
  Product23 : Product  Inputs=3
  Product24 : Product
  Producto{,3..4,6} (4 alike) : Product
  Producto{1..2,5,7..10} (7 alike) : Product  Inputs=3
  Square{,1..4} (5 alike) : Math  Operator=square  SignedPower=on  SaturateOnIntegerOverflow=on
  Sum{5,19..21,23..24} (6 alike) : Sum  Inputs=|++
  Sum2 : Sum  Inputs=-+++
  Sum22 : Sum  Inputs=|+-
  Sum9 : Sum  Inputs=|+-
  T4 : Math  Operator=pow  SignedPower=on  SaturateOnIntegerOverflow=on
  Terminator : Terminator
  Xu' : Gain  Gain=-0.075
  Yr : Gain  Gain=3
  Yr' : Gain  Gain=0.2
  Yr|r| : Gain
  Yr|v| : Gain
  Yv : Gain  Gain=0.5
  Yv' : Gain  Gain=0.9
  Yv|r| : Gain
  Yv|v| : Gain
  cte : Constant  Value=1.1
  cte1 : Constant  Value=4
  cte2 : Constant  Value=3
  rho*T : Product
  sqrt(u2+v2) : Sqrt  SaturateOnIntegerOverflow=on
  "Hydrodynamic Coefficients " : Outport  VectorParamsAs1DForOutWhenUnconnected=off
  wires:
  m/1 -> Xu'/1
  Nv'/1 -> Bus Creator/4  "N_v_dot"
  Xu'/1 -> Bus Creator/1  "X_u_dot"
  Square/1 -> Gain13/1
  Gain14/1 -> Product23/1
  Product24/1 -> Gain14/1
  Sum9/1 -> (L-LCG)3/1, (L-LCG)4/1, (L-LCG)2/1
  Square4/1 -> Producto2/3
  sqrt(u2+v2)/1 -> Producto2/2, Producto1/2
  Product20/1 -> Product23/2
  Gain13/1 -> Sum2/4
  B_hull/1 -> Producto5/2, Product22/1  "B_hull"
  Square2/1 -> Sum5/2
  Sum20/1 -> Nr'/1
  Gain12/1 -> Sum2/1
  Sum21/1 -> Gain16/1
  LCG4/1 -> Sum24/2
  Sum24/1 -> Producto10/1
  (L-LCG)4/1 -> Sum24/1
  Sum2/1 -> Product23/3
  Producto10/1 -> Gain20/1
  (L-LCG)3/1 -> Sum21/1, Sum23/1
  Producto6/1 -> Sum20/1
  Gain19/1 -> Yr|r|/1, Nr|v|/1, Nv|r|/1
  Gain16/1 -> Producto6/2
  Sum22/1 -> Producto8/2
  Producto3/1 -> Yv'/1
  Gain10/1 -> Product20/1
  cte1/1 -> LCG4/2, T4/2, (L-LCG)4/2
  cte2/1 -> (L-LCG)3/2, LCG3/2
  Product23/1 -> Yv/1
  cte/1 -> Sum2/2
  Producto8/1 -> Gain18/1
  Sum23/1 -> Producto9/1
  Gain20/1 -> Nr|r|/1
  Gain18/1 -> Nv|v|/1, Yr|v|/1, Yv|r|/1
  Yr'/1 -> Bus Creator/3  "Y_r_dot"
  Producto7/1 -> Gain17/1
  Producto9/1 -> Gain19/1
  Gain11/1 -> Sum2/3
  Square1/1 -> Producto/2
  Producto2/1 -> Nr/1
  LCG3/1 -> Sum21/2, Sum23/2
  T4/1 -> Producto5/3
  Gain40/1 -> Sum20/2
  Producto4/1 -> Yr'/1, Nv'/1
  Sum19/1 -> Gain15/1
  Square3/1 -> Sum5/1
  Sum5/1 -> sqrt(u2+v2)/1
  rho/1 -> Producto/1, Gain10/1, Producto5/1, rho*T/1  "rho"
  Abs v1/1 -> Product20/2
  Product21/1 -> Gain11/1
  Gain17/1 -> Yv|v|/1
  (L-LCG)2/1 -> Sum19/1, Sum22/1
  Producto1/1 -> Nv/1, Yr/1
  Product22/1 -> Square/1, Gain12/1
  LCG2/1 -> Sum19/2, Sum22/2
  LCG/1 -> Sum9/2, LCG2/1, LCG3/1, LCG4/1  "LCG"
  Producto/1 -> -pi*rho*T^2/1
  -pi*rho*T^2/1 -> Producto4/1, Producto3/2, Producto2/1, Producto1/1, Producto6/1
  Producto5/1 -> Gain40/1
  Gain15/1 -> Producto4/2
  rho*T/1 -> Producto9/2, Producto10/2, Producto7/3, Producto8/3
  T/1 -> Product21/2, rho*T/2, T4/1, Square1/1, Product22/2, Product24/2  "T"
  L/1 -> Producto7/1, Square4/1, Producto1/3, Producto3/1, Product21/1, Product24/1, Sum9/1  "L"
  C_d/1 -> Producto7/2, Producto8/1, Producto9/3, Producto10/3  "C_d"
  Nv/1 -> Bus Creator/15  "N_v"
  Yv|v|/1 -> Bus Creator/8  "Y_v|v|"
  Yr|r|/1 -> Bus Creator/12  "Y_r|r|"
  Yv/1 -> Bus Creator/10  "Y_v"
  Nv|v|/1 -> Bus Creator/14  "N_v|v|"
  Yr|v|/1 -> Bus Creator/11  "Y_r|v|"
  Nv|r|/1 -> Bus Creator/16  "N_v|r|"
  Yr/1 -> Bus Creator/13  "Y_r"
  Nr|r|/1 -> Bus Creator/19  "N_r|r|"
  Nr/1 -> Bus Creator/18  "N_r"
  Xu|u|/1 -> Bus Creator/7  "X_u|u|"
  Yv|r|/1 -> Bus Creator/9  "Y_v|r|"
  Nr|v|/1 -> Bus Creator/17  "N_r|v|"
  Xu/1 -> Bus Creator/6  "X_u"
  Bus Creator/1 -> "Hydrodynamic Coefficients "/1
  Nr'/1 -> Bus Creator/5  "N_r_dot"
  Yv'/1 -> Bus Creator/2  "Y_v_dot"
  Demux/1 -> Square3/1  "u"
  V local/1 -> Demux/1
  Demux/2 -> Abs v1/1, Square2/1  "v"
  Demux/3 -> Terminator/1  "r"

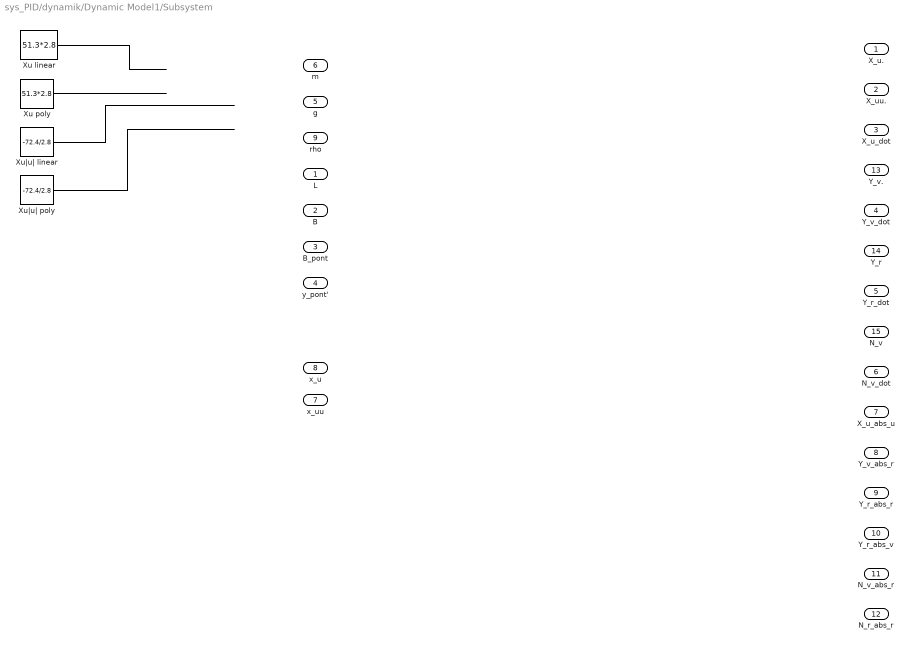
== system sys_PID/dynamik/Dynamic Model1/Subsystem ==
  L : Inport
  B : Inport  Port=2
  B_pont : Inport  Port=3
  y_pont' : Inport  Port=4
  g : Inport  Port=5
  m : Inport  Port=6
  x_uu : Inport  Port=7
  x_u : Inport  Port=8
  rho : Inport  Port=9
  Xu linear : Constant  Value=51.3*2.8
  Xu poly : Constant  Value=51.3*2.8
  Xu|u| linear : Constant  Value=-72.4/2.8
  Xu|u| poly : Constant  Value=-72.4/2.8
  X_u. : Outport
  X_uu. : Outport  Port=2
  X_u_dot : Outport  Port=3
  Y_v_dot : Outport  Port=4
  Y_r_dot : Outport  Port=5
  N_v_dot : Outport  Port=6
  X_u_abs_u : Outport  Port=7
  Y_v_abs_r : Outport  Port=8
  Y_r_abs_r : Outport  Port=9
  Y_r_abs_v : Outport  Port=10
  N_v_abs_r : Outport  Port=11
  N_r_abs_r : Outport  Port=12
  Y_v. : Outport  Port=13
  Y_r : Outport  Port=14
  N_v : Outport  Port=15
  wires:
  Xu|u| linear/1 -> ?
  Xu|u| poly/1 -> ?
  Xu poly/1 -> ?
  Xu linear/1 -> ?

== system sys_PID/dynamik/Dynamic Model1/Subsystem5 ==
  psi : Inport
  " J(n)" : sharedutil/Create 3x3 Matrix  aMode=aMode
      settings: SourceProductBaseCode=AE,PW,DR,MT,UV,VE
  Constant1 : Constant
  Constant2 : Constant  Value=0
  Gain9 : Gain  Gain=-1
  Selector : Selector  InputPortWidth=3  IndexOptions=Index vector (dialog)  Indices=3  OutputSizes=1
  Trigonometric Function : Trigonometry
  Trigonometric Function1 : Trigonometry  Operator=cos
  J(n) : Outport  VectorParamsAs1DForOutWhenUnconnected=off
  wires:
  Gain9/1 -> " J(n)"/2
  Trigonometric Function1/1 -> " J(n)"/5, " J(n)"/1
  Trigonometric Function/1 -> " J(n)"/4, Gain9/1
  Constant1/1 -> " J(n)"/9
  psi/1 -> Selector/1
  " J(n)"/1 -> J(n)/1
  Constant2/1 -> " J(n)"/8, " J(n)"/7, " J(n)"/6, " J(n)"/3
  Selector/1 -> Trigonometric Function1/1, Trigonometric Function/1

== system sys_PID/dynamik/Dynamic Model1/Construct Matrices/M ==
  Hydrodynamic coefficients : Inport
  m1 : Inport  Port=2
  x_g : Inport  Port=3
  y_g : Inport  Port=4
  I_z1 : Inport  Port=5
  Bus Selector : BusSelector  OutputSignals=X_u_dot,Y_r_dot,N_v_dot,Y_v_dot,N_r_dot
  M-matrice : MATLAB Function  TreatAsAtomicUnit=on
  Out_M : Outport
  wires:
  Hydrodynamic coefficients/1 -> Bus Selector/1
  m1/1 -> M-matrice/1(m)
  I_z1/1 -> M-matrice/4(I_z)
  y_g/1 -> M-matrice/3(y_g)
  x_g/1 -> M-matrice/2(x_g)
  M-matrice/1(M_out) -> Out_M/1
  Bus Selector/1 -> M-matrice/5(Xu_dot)  "<X_u_dot>"
  Bus Selector/2 -> M-matrice/7(Yr_dot)  "<Y_r_dot>"
  Bus Selector/4 -> M-matrice/6(Yv_dot)  "<Y_v_dot>"
  Bus Selector/5 -> M-matrice/8(Nr_dot)  "<N_r_dot>"
  Bus Selector/3 -> M-matrice/9(Nv_dot)  "<N_v_dot>"

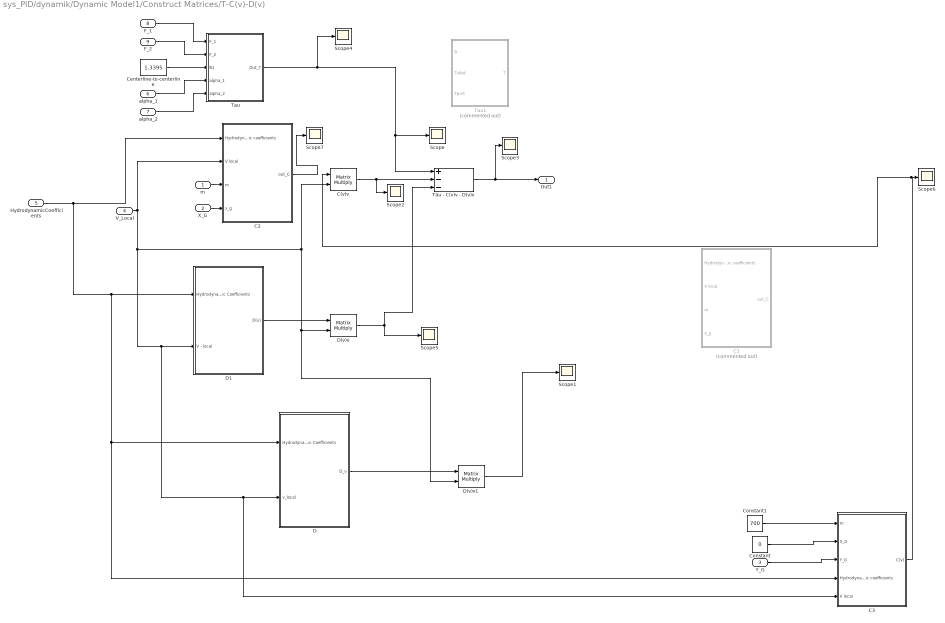
== system sys_PID/dynamik/Dynamic Model1/Construct Matrices/T-C(v)-D(v) ==
  m : Inport
  X_G : Inport  Port=2
  Y_G : Inport  Port=3
  V_Local : Inport  Port=4
  HydrodynamicCoefficients : Inport  Port=5
  alpha_1 : Inport  Port=6
  alpha_2 : Inport  Port=7
  F_1 : Inport  Port=8
  F_2 : Inport  Port=9
  C(v)v : Product  Multiplication=Matrix(*)
  C1 : Subsystem  Commented=on
  C2 : Subsystem
  C3 : Subsystem
  Centerline-to-centerline : Constant  Value=1.3395
  Constant : Constant  Value=0
  Constant1 : Constant  Value=700
  D : Subsystem
  D(v)v : Product  Multiplication=Matrix(*)
  D(v)v1 : Product  Multiplication=Matrix(*)
  D1 : Subsystem
  Scope{,1..7} (8 alike) : Scope
  Tau : Subsystem
  Tau - C(v)v - D(v)v : Sum  Inputs=+--
  Tau1 : Subsystem  Commented=on
  Out1 : Outport  VectorParamsAs1DForOutWhenUnconnected=off
  wires:
  V_Local/1 -> C2/2(V local), C3/5(V local), D/2(v_local), D1/2(V - local), D(v)v1/2, D(v)v/2, C(v)v/2
  Tau - C(v)v - D(v)v/1 -> Scope3/1, Out1/1
  HydrodynamicCoefficients/1 -> C2/1(Hydrodynamic coefficients), D/1(Hydrodynamic Coefficients), C3/4(Hydrodynamic coefficients), D1/1(Hydrodynamic Coefficients)
  Centerline-to-centerline/1 -> Tau/3(B1)
  F_2/1 -> Tau/2(F_2)
  F_1/1 -> Tau/1(F_1)
  m/1 -> C2/3(m)
  X_G/1 -> C2/4(x_g)
  Y_G/1 -> C3/3(Y_G)
  C2/1(out_C) -> Scope7/1
  D1/1(D(v)) -> D(v)v/1
  C(v)v/1 -> Scope2/1, Tau - C(v)v - D(v)v/2
  alpha_1/1 -> Tau/4(alpha_1)
  alpha_2/1 -> Tau/5(alpha_2)
  D/1(D_v) -> D(v)v1/1
  D(v)v/1 -> Tau - C(v)v - D(v)v/3, Scope5/1
  D(v)v1/1 -> Scope1/1
  Tau/1(Out_T) -> Scope4/1, Scope/1, Tau - C(v)v - D(v)v/1
  Constant/1 -> C3/2(X_G)
  Constant1/1 -> C3/1(m)
  C3/1(C(v)) -> C(v)v/1, Scope6/1

== system sys_PID/dynamik/Dynamic Model1/Construct Matrices/T-C(v)-D(v)/C1 ==
  Hydrodynamic coefficients : Inport
  V local : Inport  Port=2
  m : Inport  Port=3
  x_g : Inport  Port=4
  Demux : Demux  Outputs=19
  Demux1 : Demux  Outputs=3
  MATLAB Function : MATLAB Function  TreatAsAtomicUnit=on
  out_C : Outport
  wires:
  Hydrodynamic coefficients/1 -> Demux/1
  V local/1 -> Demux1/1
  MATLAB Function/1(y) -> out_C/1
  Demux1/1 -> MATLAB Function/2(u)  "u"
  Demux1/2 -> MATLAB Function/1(v)  "v"
  Demux1/3 -> MATLAB Function/3(r)  "r"
  Demux/1 -> MATLAB Function/6(Xu_dot)
  Demux/2 -> MATLAB Function/7(Yv_dot)
  Demux/3 -> MATLAB Function/8(Yr_dot)
  x_g/1 -> MATLAB Function/5(x_g)
  m/1 -> MATLAB Function/4(m)

== system sys_PID/dynamik/Dynamic Model1/Construct Matrices/T-C(v)-D(v)/C2 ==
  Hydrodynamic coefficients : Inport
  V local : Inport  Port=2
  m : Inport  Port=3
  x_g : Inport  Port=4
  Demux : Demux  Outputs=19
  Demux1 : Demux  Outputs=3
  MATLAB Function : MATLAB Function  TreatAsAtomicUnit=on
  out_C : Outport
  wires:
  Hydrodynamic coefficients/1 -> Demux/1
  V local/1 -> Demux1/1
  MATLAB Function/1(y) -> out_C/1
  Demux1/1 -> MATLAB Function/2(u)  "u"
  Demux1/2 -> MATLAB Function/1(v)  "v"
  Demux1/3 -> MATLAB Function/3(r)  "r"
  Demux/1 -> MATLAB Function/6(Xu_dot)
  Demux/2 -> MATLAB Function/7(Yv_dot)
  Demux/3 -> MATLAB Function/8(Yr_dot)
  x_g/1 -> MATLAB Function/5(x_g)
  m/1 -> MATLAB Function/4(m)

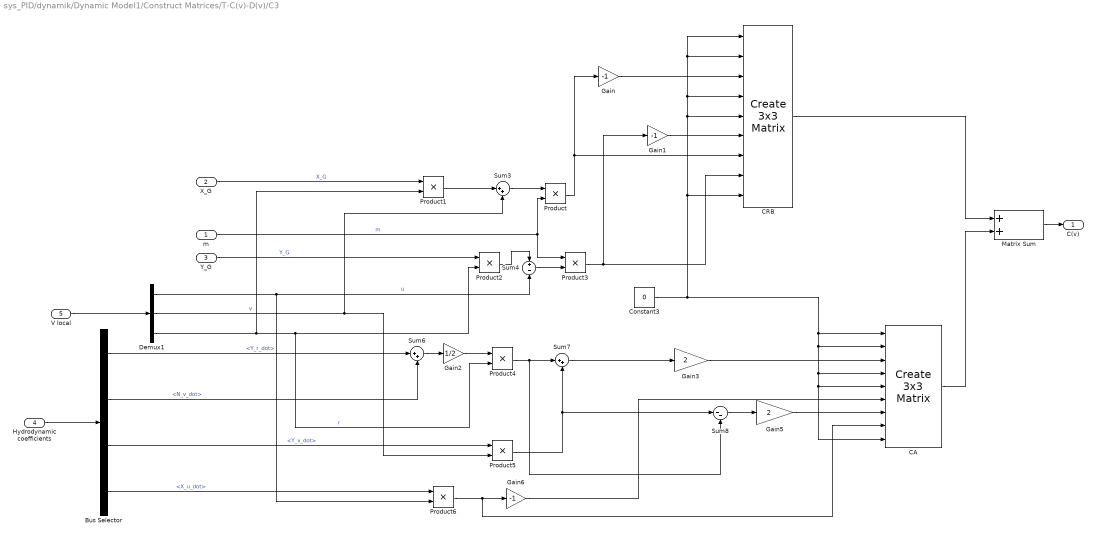
== system sys_PID/dynamik/Dynamic Model1/Construct Matrices/T-C(v)-D(v)/C3 ==
  m : Inport
  X_G : Inport  Port=2
  Y_G : Inport  Port=3
  Hydrodynamic coefficients : Inport  Port=4
  V local : Inport  Port=5
  " CRB" : sharedutil/Create 3x3 Matrix  aMode=aMode
      settings: SourceProductBaseCode=AE,PW,DR,MT,UV,VE
  Bus Selector : BusSelector  OutputSignals=Y_r_dot,N_v_dot,Y_v_dot,X_u_dot
  CA : sharedutil/Create 3x3 Matrix  aMode=aMode
      settings: SourceProductBaseCode=AE,PW,DR,MT,UV,VE
  Constant3 : Constant  Value=0
  Demux1 : Demux  Outputs=3
  Gain : Gain  Gain=-1
  Gain1 : Gain  Gain=-1
  Gain2 : Gain  Gain=1/2
  Gain3 : Gain  Gain=2
  Gain5 : Gain  Gain=2
  Gain6 : Gain  Gain=-1
  Matrix Sum : Sum
  Product{,1..6} (7 alike) : Product
  Sum3 : Sum  Inputs=|++
  Sum4 : Sum  Inputs=+-
  Sum6 : Sum  Inputs=|++
  Sum7 : Sum  Inputs=|++
  Sum8 : Sum  Inputs=|--
  C(v) : Outport  VectorParamsAs1DForOutWhenUnconnected=off
  wires:
  Bus Selector/1 -> Sum6/1  "<Y_r_dot>"
  Demux1/3 -> Product1/2, Product2/2, Product4/2  "r"
  Gain2/1 -> Product4/1
  CA/1 -> Matrix Sum/2
  Gain/1 -> " CRB"/3
  Bus Selector/2 -> Sum6/2  "<N_v_dot>"
  Sum3/1 -> Product/1
  Sum8/1 -> Gain5/1
  Product2/1 -> Sum4/1
  Sum6/1 -> Gain2/1
  Product5/1 -> Sum7/2, Sum8/1
  Gain1/1 -> " CRB"/6
  Product1/1 -> Sum3/1
  Y_G/1 -> Product2/1  "Y_G"
  Matrix Sum/1 -> C(v)/1
  Gain3/1 -> CA/3
  Gain6/1 -> CA/6
  Product6/1 -> Gain6/1, CA/8
  Demux1/2 -> Sum3/2, Product5/2  "v"
  Product4/1 -> Sum7/1, Sum8/2
  Product3/1 -> " CRB"/8, Gain1/1
  Gain5/1 -> CA/7
  " CRB"/1 -> Matrix Sum/1
  X_G/1 -> Product1/1  "X_G"
  Sum7/1 -> Gain3/1
  Product/1 -> " CRB"/7, Gain/1
  m/1 -> Product/2, Product3/1  "m"
  Constant3/1 -> " CRB"/5, " CRB"/4, " CRB"/2, " CRB"/1, " CRB"/9, CA/4, CA/5, CA/9, CA/2, CA/1
  Hydrodynamic coefficients/1 -> Bus Selector/1
  Bus Selector/4 -> Product6/1  "<X_u_dot>"
  Bus Selector/3 -> Product5/1  "<Y_v_dot>"
  Demux1/1 -> Sum4/2, Product6/2  "u"
  V local/1 -> Demux1/1
  Sum4/1 -> Product3/2

== system sys_PID/dynamik/Dynamic Model1/Construct Matrices/T-C(v)-D(v)/D ==
  Hydrodynamic Coefficients : Inport
  v_local : Inport  Port=2
  Bus Selector : BusSelector  OutputSignals=X_u,Y_v,Y_r,X_u|u|,Y_v|v|,Y_v|r|,Y_r|v|,N_v,N_r,Y_r|r|,N_v|v|,N_v|r|,N_r|r|,N_r|v|
  Demux1 : Demux  Outputs=3
  MATLAB Function : MATLAB Function  TreatAsAtomicUnit=on
  D_v : Outport
  wires:
  Hydrodynamic Coefficients/1 -> Bus Selector/1
  Demux1/3 -> MATLAB Function/3(r)
  MATLAB Function/1(D_v) -> D_v/1
  v_local/1 -> Demux1/1
  Bus Selector/1 -> MATLAB Function/4(X_u)  "<X_u>"
  Bus Selector/2 -> MATLAB Function/5(Y_v)  "<Y_v>"
  Bus Selector/14 -> MATLAB Function/16(N_r_abs_v)  "<N_r|v|>"
  Bus Selector/13 -> MATLAB Function/15(N_r_abs_r)  "<N_r|r|>"
  Bus Selector/12 -> ?  "<N_v|r|>"
  Bus Selector/11 -> MATLAB Function/14(N_v_abs_v)  "<N_v|v|>"
  Bus Selector/10 -> MATLAB Function/13(Y_r_abs_r)  "<Y_r|r|>"
  Bus Selector/9 -> MATLAB Function/7(N_r)  "<N_r>"
  Bus Selector/8 -> MATLAB Function/8(N_v)  "<N_v>"
  Bus Selector/7 -> MATLAB Function/12(Y_r_abs_v)  "<Y_r|v|>"
  Bus Selector/6 -> MATLAB Function/10(Y_v_abs_r)  "<Y_v|r|>"
  Bus Selector/5 -> MATLAB Function/9(Y_v_abs_v)  "<Y_v|v|>"
  Bus Selector/4 -> MATLAB Function/11(x_u_abs_u)  "<X_u|u|>"
  Bus Selector/3 -> MATLAB Function/6(Y_r)  "<Y_r>"
  Demux1/1 -> MATLAB Function/2(u)
  Demux1/2 -> MATLAB Function/1(v)

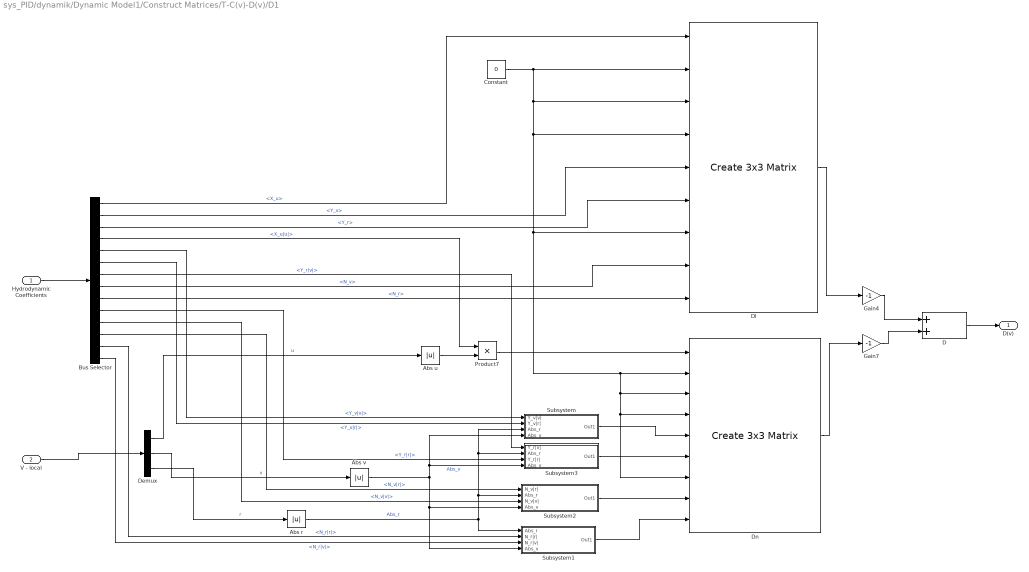
== system sys_PID/dynamik/Dynamic Model1/Construct Matrices/T-C(v)-D(v)/D1 ==
  Hydrodynamic Coefficients : Inport
  V - local : Inport  Port=2
  Abs r : Abs
  Abs u : Abs
  Abs v : Abs
  Bus Selector : BusSelector  OutputSignals=X_u,Y_v,Y_r,X_u|u|,Y_v|v|,Y_v|r|,Y_r|v|,N_v,N_r,Y_r|r|,N_v|v|,N_v|r|,N_r|r|,N_r|v|
  Constant : Constant  Value=0
  D : Sum
  Demux : Demux  Outputs=3
  Dl : sharedutil/Create 3x3 Matrix  aMode=aMode
      settings: SourceProductBaseCode=AE,PW,DR,MT,UV,VE
  Dn : sharedutil/Create 3x3 Matrix  aMode=aMode
      settings: SourceProductBaseCode=AE,PW,DR,MT,UV,VE
  Gain4 : Gain  Gain=-1
  Gain7 : Gain  Gain=-1
  Product7 : Product
  Subsystem : Subsystem
  Subsystem1 : Subsystem
  Subsystem2 : Subsystem
  Subsystem3 : Subsystem
  D(v) : Outport  VectorParamsAs1DForOutWhenUnconnected=off
  wires:
  Constant/1 -> Dn/7, Dn/4, Dn/3, Dn/2, Dl/7, Dl/4, Dl/3, Dl/2
  Abs u/1 -> Product7/2
  Abs r/1 -> Subsystem/3(Abs_r), Subsystem3/2("Abs_r "), Subsystem2/2(Abs_r), Subsystem1/1(Abs_r)  "Abs_r"
  Product7/1 -> Dn/1
  Abs v/1 -> Subsystem/4("Abs_v "), Subsystem3/4(Abs_v), Subsystem1/4(Abs_v), Subsystem2/4(Abs_v)  "Abs_v"
  Gain7/1 -> D/2
  Gain4/1 -> D/1
  Dl/1 -> Gain4/1
  Dn/1 -> Gain7/1
  D/1 -> D(v)/1
  Subsystem/1(Out1) -> Dn/5
  Subsystem1/1(Out1) -> Dn/9
  Subsystem2/1(Out1) -> Dn/8
  Subsystem3/1(Out1) -> Dn/6
  Hydrodynamic Coefficients/1 -> Bus Selector/1
  Bus Selector/5 -> Subsystem/1("Y_v|v| ")  "<Y_v|v|>"
  Bus Selector/6 -> Subsystem/2(Y_v|r|)  "<Y_v|r|>"
  Bus Selector/2 -> Dl/5  "<Y_v>"
  Bus Selector/7 -> Subsystem3/1(Y_r|v|)  "<Y_r|v|>"
  Bus Selector/10 -> Subsystem3/3(Y_r|r|)  "<Y_r|r|>"
  Bus Selector/11 -> Subsystem2/3(N_v|v|)  "<N_v|v|>"
  Bus Selector/8 -> Dl/8  "<N_v>"
  Bus Selector/12 -> Subsystem2/1(N_v|r|)  "<N_v|r|>"
  Bus Selector/14 -> Subsystem1/3(N_r|v|)  "<N_r|v|>"
  Bus Selector/9 -> Dl/9  "<N_r>"
  Bus Selector/13 -> Subsystem1/2(N_r|r|)  "<N_r|r|>"
  Bus Selector/1 -> Dl/1  "<X_u>"
  Bus Selector/4 -> Product7/1  "<X_u|u|>"
  Bus Selector/3 -> Dl/6  "<Y_r>"
  Demux/1 -> Abs u/1  "u"
  Demux/2 -> Abs v/1  "v"
  Demux/3 -> Abs r/1  "r"
  V - local/1 -> Demux/1

== system sys_PID/dynamik/Dynamic Model1/Construct Matrices/T-C(v)-D(v)/Tau ==
  F_1 : Inport
  F_2 : Inport  Port=2
  B1 : Inport  Port=3
  alpha_1 : Inport  Port=4
  alpha_2 : Inport  Port=5
  MATLAB Function : MATLAB Function  TreatAsAtomicUnit=on
  MATLAB Function1 : MATLAB Function  Commented=on  TreatAsAtomicUnit=on
  Out_T : Outport
  wires:
  F_1/1 -> MATLAB Function/1(F_1)
  MATLAB Function/1(y) -> Out_T/1
  B1/1 -> MATLAB Function/5(d)
  F_2/1 -> MATLAB Function/2(F_2)
  alpha_1/1 -> MATLAB Function/3(alpha_1)
  alpha_2/1 -> MATLAB Function/4(alpha_2)

== system sys_PID/dynamik/Dynamic Model1/Construct Matrices/T-C(v)-D(v)/Tau1 ==
  B : Inport
  Tstbd : Inport  Port=2
  Tport : Inport  Port=3
  Correction factor : Gain
  Mux : Mux  Inputs=3
  Product25 : Product
  Sum : Sum  Inputs=|++
  Sum1 : Sum  Inputs=|+-
  Ty : Constant  Value=0
  Tz : Gain  Gain=1/2
  T : Outport  VectorParamsAs1DForOutWhenUnconnected=off
  wires:
  Product25/1 -> Tz/1
  Tz/1 -> Mux/3  "Tz"
  Mux/1 -> T/1  "T"
  B/1 -> Product25/1  "B"
  Sum1/1 -> Product25/2
  Ty/1 -> Mux/2  "Ty"
  Tstbd/1 -> Correction factor/1  "Tstbd"
  Tport/1 -> Sum/1, Sum1/1  "Tport"
  Sum/1 -> Mux/1
  Correction factor/1 -> Sum/2, Sum1/2  "Tstbd"

== system sys_PID/dynamik/Dynamic Model1/Construct Matrices/T-C(v)-D(v)/D1/Subsystem ==
  "Y_v|v| " : Inport
  Y_v|r| : Inport  Port=2
  Abs_r : Inport  Port=3
  "Abs_v " : Inport  Port=4
  Product8 : Product
  Product9 : Product
  Sum10 : Sum  Inputs=|++
  Out1 : Outport  VectorParamsAs1DForOutWhenUnconnected=off
  wires:
  Y_v|r|/1 -> Product9/1
  Abs_r/1 -> Product9/2
  Product9/1 -> Sum10/2
  "Y_v|v| "/1 -> Product8/1
  Product8/1 -> Sum10/1
  "Abs_v "/1 -> Product8/2
  Sum10/1 -> Out1/1

== system sys_PID/dynamik/Dynamic Model1/Construct Matrices/T-C(v)-D(v)/D1/Subsystem1 ==
  Abs_r : Inport
  N_r|r| : Inport  Port=2
  N_r|v| : Inport  Port=3
  Abs_v : Inport  Port=4
  Product14 : Product
  Product15 : Product
  Sum13 : Sum  Inputs=|++
  Out1 : Outport  VectorParamsAs1DForOutWhenUnconnected=off
  wires:
  Product15/1 -> Sum13/1
  Sum13/1 -> Out1/1
  N_r|v|/1 -> Product14/1
  Product14/1 -> Sum13/2
  Abs_r/1 -> Product15/2
  N_r|r|/1 -> Product15/1
  Abs_v/1 -> Product14/2

== system sys_PID/dynamik/Dynamic Model1/Construct Matrices/T-C(v)-D(v)/D1/Subsystem2 ==
  N_v|r| : Inport
  Abs_r : Inport  Port=2
  N_v|v| : Inport  Port=3
  Abs_v : Inport  Port=4
  Product12 : Product
  Product13 : Product
  Sum12 : Sum  Inputs=|++
  Out1 : Outport  VectorParamsAs1DForOutWhenUnconnected=off
  wires:
  Sum12/1 -> Out1/1
  Product13/1 -> Sum12/1
  N_v|v|/1 -> Product12/1
  Product12/1 -> Sum12/2
  Abs_r/1 -> Product13/2
  Abs_v/1 -> Product12/2
  N_v|r|/1 -> Product13/1

== system sys_PID/dynamik/Dynamic Model1/Construct Matrices/T-C(v)-D(v)/D1/Subsystem3 ==
  Y_r|v| : Inport
  "Abs_r " : Inport  Port=2
  Y_r|r| : Inport  Port=3
  Abs_v : Inport  Port=4
  Product10 : Product
  Product11 : Product
  Sum11 : Sum  Inputs=|++
  Out1 : Outport  VectorParamsAs1DForOutWhenUnconnected=off
  wires:
  Product11/1 -> Sum11/2
  Product10/1 -> Sum11/1
  Sum11/1 -> Out1/1
  Y_r|v|/1 -> Product10/1
  "Abs_r "/1 -> Product11/2
  Y_r|r|/1 -> Product11/1
  Abs_v/1 -> Product10/2
